simulink model "Flexible_joints_manip_simulink_Final_working"  (R2018b)
settings: Solver=FixedStepAuto  StartTime=0.0  StopTime=10  FixedStep=0.00001  MaxStep=0.01  MinStep=0.0000001  RelTol=1e-3
settings Model: Creator=ahmed  LastModifiedBy=ahmed
settings SolverCC: MaxConsecutiveMinStep=10

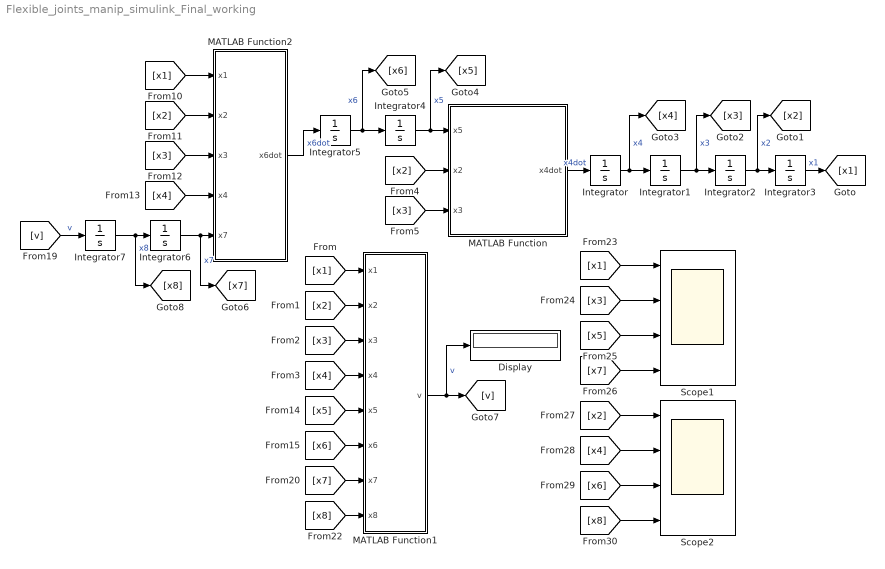
== system Flexible_joints_manip_simulink_Final_working ==
  Display : Display
      settings: Decimation=3
  Integrator{,2..3,5..7} (6 alike) : Integrator
  Integrator1 : Integrator  InitialCondition=pi/4
  Integrator4 : Integrator  InitialCondition=pi/4
  MATLAB Function : MATLAB Function  TreatAsAtomicUnit=on
  MATLAB Function1 : MATLAB Function  TreatAsAtomicUnit=on
  MATLAB Function2 : MATLAB Function  TreatAsAtomicUnit=on
  Scope1 : Scope  NumInputPorts=4
  Scope2 : Scope  NumInputPorts=4
  wires:
  MATLAB Function/1(x4dot) -> Integrator/1  "x4dot"
  Integrator/1 -> Integrator1/1, [x4]  "x4"
  Integrator2/1 -> Integrator3/1, [x2]  "x2"
  [x2] -> MATLAB Function/2(x2)
  [x3] -> MATLAB Function/3(x3)
  [x4] -> MATLAB Function1/4(x4)
  [x2] -> MATLAB Function1/2(x2)
  Integrator5/1 -> [x6], Integrator4/1  "x6"
  MATLAB Function2/1(x6dot) -> Integrator5/1  "x6dot"
  [x6] -> MATLAB Function1/6(x6)
  [x1] -> MATLAB Function2/1(x1)
  [x2] -> MATLAB Function2/2(x2)
  [x3] -> MATLAB Function2/3(x3)
  [x4] -> MATLAB Function2/4(x4)
  MATLAB Function1/1(v) -> Display/1, [v]  "v"
  [v] -> Integrator7/1  "v"
  Integrator7/1 -> [x8], Integrator6/1  "x8"
  [x8] -> MATLAB Function1/8(x8)
  [x1] -> Scope1/1
  [x3] -> Scope1/2
  [x5] -> Scope1/3
  [x7] -> Scope1/4
  [x2] -> Scope2/1
  [x4] -> Scope2/2
  [x6] -> Scope2/3
  [x8] -> Scope2/4
  Integrator3/1 -> [x1]  "x1"
  Integrator1/1 -> Integrator2/1, [x3]  "x3"
  Integrator4/1 -> MATLAB Function/1(x5), [x5]  "x5"
  Integrator6/1 -> [x7], MATLAB Function2/5(x7)  "x7"
  [x1] -> MATLAB Function1/1(x1)
  [x3] -> MATLAB Function1/3(x3)
  [x5] -> MATLAB Function1/5(x5)
  [x7] -> MATLAB Function1/7(x7)

== matlab function Flexible_joints_manip_simulink_Final_working/MATLAB Function1 ==
  data: x1 input; v output; x2 input; x3 input; x4 input; x5 input; x6 input; x7 input; x8 input
function v = fcn(x1,x2,x3,x4,x5,x6,x7,x8)

p1 = 1.5; p2 = 0.5; p3 = 2; p4 = 0.2; p5 = 1; p6 = 1; p7 = 50;
k1 = 100; k2 = 200;

e2 = x2 + x1;
e3 = x3 + 2*e2;
e4 = x4 + 3*e3 - e2 - 2*x1;
e5 = (k2/p3)*x5 + 4*e4 - (3+(k2/p3))*e3 - (4-2*(k2/p3))*e2 + 3*x1 ...
     - (p7/p3)*cos(e3-2*e2) ...
     - (p2/(2*p3))*(e2-x1)^2*sin(2*(e3-2*e2));
e6 = (k2/p3)*x6 + 5*e5 - (6+(k2/p3))*e4 - (5-3*(k2/p3))*e3 ...
     + (10-(k2/p3))*e2 + (1-2*(k2/p3))*x1 ...
     + (p7/p3)*(e4-3*e3+e2+2*x1)*sin(e3-2*e2) ...
     - (p2/p3)*(e2-x1)*(e3-2*e2)*sin(2*(e3-2*e2)) ...
     - (p2/p3)*(e2-x1)^2*(e4-3*e3+e2+2*x1)*cos(2*(e3-2*e2));

phi = (k2*p2/(p3*p4))*(e2-x1)*(e4-3*e3+e2+2*x1)*sin(2*(e3-2*e2)) ...
     - (k2*p2/(p3*p4))*(e3-2*e2)*cos(e3-2*e2)^2 ...
     + (p7/p3)*(e4-3*e3+e2+2*x1)^2*cos(e3-2*e2) ...
     + (p7/p3)*(e5-4*e4+3*e3+4*e2-3*x1)*sin(e3-2*e2) ...
     - (2*p2/p3)*(e2-x1)*(e3-2*e2)*(e4-3*e3+e2+2*x1)*cos(2*(e3-2*e2)) ...
     - (p2/p3)*(e2-x1)*(e4-3*e3+e2+2*x1)*sin(2*(e3-2*e2)) ...
     - (p2/p3)*(e3-2*e2)^2*sin(2*(e3-2*e2)) ...
     + (2*p2/p3)*(e2-x1)^2*(e4-3*e3+e2+2*x1)^2*sin(2*(e3-2*e2)) ...
     - (p2/p3)*(e2-x1)^2*(e5-4*e4+3*e3+4*e2-3*x1)*cos(2*(e3-2*e2)) ...
     - (2*p2/p3)*(e2-x1)*(e3-2*e2)*(e4-3*e3+e2+2*x1)*cos(2*(e3-2*e2));

e7 = (k1*k2/(p3*p4))*x7 + 6*e6 - (10+(k2/p3))*e5 - (4-4*(k2/p3))*e4 ...
     + (21-3*(k2/p3)-(p1*k2/(p3*p4)))*e3 ...
     - (4+4*(k2/p3)-2*(p1*k2/(p3*p4)))*e2 ...
     - (11-3*(k2/p3)+(k1*k2/(p3*p4)))*x1 ...
     + phi;
 
phidot = -(k2*p2/(p3*p4))*(e4-3*e3+e2+2*x1)*cos(e3-2*e2)^2 ...
     - (p7/p3)*(e4-3*e3+e2+2*x1)^3*sin(e3-2*e2) ...
     + (p7/p3)*(e6-5*e5+6*e4+5*e3-10*e2-x1)*sin(e3-2*e2) ...
     + (3*p7/p3)*(e4-3*e3+e2+2*x1)*(e5-4*e4+3*e3+4*e2-3*x1)*cos(e3-2*e2) ...
     + ((2*k2*p2-3*p4*p2)/(p3*p4))*(e3-2*e2)*(e4-3*e3+e2+2*x1)*sin(2*(e3-2*e2)) ...
     + ((k2*p2-p4*p2)/(p3*p4))*(e2-x1)*(e5-4*e4+3*e3+4*e2-3*x1)*sin(2*(e3-2*e2)) ...
     + (12*p2/p3)*(e2-x1)*(e3-2*e2)*(e4-3*e3+e2+2*x1)^2*sin(2*(e3-2*e2)) ...
     + (6*p2/p3)*(e2-x1)^2*(e4-3*e3+e2+2*x1)*(e5-4*e4+3*e3+4*e2-3*x1)*sin(2*(e3-2*e2)) ...
     + (4*p2/p3)*(e2-x1)^2*(e4-3*e3+e2+2*x1)^3*cos(2*(e3-2*e2)) ...
     - (p2/p3)*(e2-x1)^2*(e6-5*e5+6*e4+5*e3-10*e2-x1)*cos(2*(e3-2*e2)) ...
     + ((2*k2*p2-6*p4*p2)/(p3*p4))*(e2-x1)*(e4-3*e3+e2+2*x1)^2*cos(2*(e3-2*e2)) ...
     - (6*p2/p3)*(e2-x1)*(e3-2*e2)*(e5-4*e4+3*e3+4*e2-3*x1)*cos(2*(e3-2*e2)) ...
     - (6*p2/p3)*(e3-2*e2)^2*(e4-3*e3+e2+2*x1)*cos(2*(e3-2*e2));

e8 = (k1*k2/(p3*p4))*x8 + 7*e7 - (15+(k2/p3))*e6 + 5*(k2/p3)*e5 ...
     + (35-6*(k2/p3)-(p1*k2/(p3*p4)))*e4 ...
     - (21+5*(k2/p3)-3*(p1*k2/(p3*p4)))*e3 ...
     - (28-10*(k2/p3)+(p1*k2/(p3*p4))+(k1*k2/(p3*p4)))*e2 ...
     + (15+(k2/p3)-2*(p1*k2/(p3*p4))+(k1*k2/(p3*p4)))*x1 ...
     + phidot;

phiddot = -(k2*p2/(p3*p4))*(e5-4*e4+3*e3+4*e2-3*x1)*cos(e3-2*e2)^2 ...
     - (p7/p3)*(e4-3*e3+e2+2*x1)^4*cos(e3-2*e2) ...
     + (3*p7/p3)*(e5-4*e4+3*e3+4*e2-3*x1)^2*cos(e3-2*e2) ...
     + (4*p7/p3)*(e4-3*e3+e2+2*x1)*(e6-5*e5+6*e4+5*e3-10*e2-x1)*cos(e3-2*e2) ...
     - (6*p7/p3)*(e4-3*e3+e2+2*x1)^2*(e5-4*e4+3*e3+4*e2-3*x1)*sin(e3-2*e2) ...
     + (p7/p3)*(e7-6*e6+10*e5+4*e4-21*e3+4*e2+11*x1)*sin(e3-2*e2) ...
     + ((3*k2*p2-3*p4*p2)/(p3*p4))*(e4-3*e3+e2+2*x1)^2*sin(2*(e3-2*e2)) ...
     + ((3*k2*p2-4*p4*p2)/(p3*p4))*(e3-2*e2)*(e5-4*e4+3*e3+4*e2-3*x1)*sin(2*(e3-2*e2)) ...
     + ((6*k2*p2-24*p4*p2)/(p3*p4))*(e3-2*e2)*(e4-3*e3+e2+2*x1)^2*cos(2*(e3-2*e2)) ...
     + ((k2*p2-p4*p2)/(p3*p4))*(e2-x1)*(e6-5*e5+6*e4+5*e3-10*e2-x1)*sin(2*(e3-2*e2)) ...
     + (48*p2/p3)*(e2-x1)*(e3-2*e2)*(e4-3*e3+e2+2*x1)*(e5-4*e4+3*e3+4*e2-3*x1)*sin(2*(e3-2*e2)) ...
     - ((4*k2*p2-24*p4*p2)/(p3*p4))*(e2-x1)*(e4-3*e3+e2+2*x1)^3*sin(2*(e3-2*e2)) ...
     + (24*p2/p3)*(e3-2*e2)^2*(e4-3*e3+e2+2*x1)^2*sin(2*(e3-2*e2)) ...
     + (8*p2/p3)*(e2-x1)^2*(e4-3*e3+e2+2*x1)*(e6-5*e5+6*e4+5*e3-10*e2-x1)*sin(2*(e3-2*e2)) ...
     + (6*p2/p3)*(e2-x1)^2*(e5-4*e4+3*e3+4*e2-3*x1)^2*sin(2*(e3-2*e2)) ...
     - (8*p2/p3)*(e2-x1)^2*(e4-3*e3+e2+2*x1)^4*sin(2*(e3-2*e2)) ...
     + ((6*k2*p2-20*p4*p2)/(p3*p4))*(e2-x1)*(e4-3*e3+e2+2*x1)*(e5-4*e4+3*e3+4*e2-3*x1)*cos(2*(e3-2*e2)) ...
     + (32*p2/p3)*(e2-x1)*(e3-2*e2)*(e4-3*e3+e2+2*x1)^3*cos(2*(e3-2*e2)) ...
     + (24*p2/p3)*(e2-x1)^2*(e4-3*e3+e2+2*x1)^2*(e5-4*e4+3*e3+4*e2-3*x1)*cos(2*(e3-2*e2)) ...
     - (p2/p3)*(e2-x1)^2*(e7-6*e6+10*e5+4*e4-21*e3+4*e2+11*x1)*cos(2*(e3-2*e2)) ...
     - (8*p2/p3)*(e2-x1)*(e3-2*e2)*(e6-5*e5+6*e4+5*e3-10*e2-x1)*cos(2*(e3-2*e2)) ...
     - (12*p2/p3)*(e3-2*e2)^2*(e5-4*e4+3*e3+4*e2-3*x1)*cos(2*(e3-2*e2));

v = (p3*p4/(k1*k2))*(-8*e8 + (21+(k2/p3))*e7 - (8+6*(k2/p3))*e6 ...
    - (50-10*(k2/p3)-(p1*k2/(p3*p4)))*e5 ...
    + (56+4*(k2/p3)-4*(p1*k2/(p3*p4)))*e4 ...
    + (42-21*(k2/p3)+3*(p1*k2/(p3*p4))+(k1*k2/(p3*p4)))*e3 ...
    - (64-4*(k2/p3)-4*(p1*k2/(p3*p4))+2*(k1*k2/(p3*p4)))*e2 ...
    - (13-11*(k2/p3)+3*(p1*k2/(p3*p4)))*x1 ...
    - phiddot);
% - phiddot); minus is the correct one mathematically!

== matlab function Flexible_joints_manip_simulink_Final_working/MATLAB Function ==
  data: x5 input; x4dot output; x2 input; x3 input
function x4dot = fcn(x5,x2,x3)

p1 = 1.5; p2 = 0.5; p3 = 2; p4 = 0.2; p5 = 1; p6 = 1; p7 = 50;
k1 = 100; k2 = 200;

x4dot = (k2/p3)*x5 - (1/(2*p3))*(p2*x2^2*sin(2*x3) + 2*k2*x3 + 2*p7*cos(x3));

== matlab function Flexible_joints_manip_simulink_Final_working/MATLAB Function2 ==
  data: x1 input; x2 input; x3 input; x4 input; x7 input; x6dot output
function x6dot = fcn(x1,x2,x3,x4,x7)

p1 = 1.5; p2 = 0.5; p3 = 2; p4 = 0.2; p5 = 1; p6 = 1; p7 = 50;
k1 = 100; k2 = 200;

x6dot = (k1/p4)*x7 - (1/p4)*(-p2*x2*x4*sin(2*x3) + k1*x1 + p1*x3 + p2*x3*cos(x3)^2);
